simulink model "P2_SIL_Model_Diag"  (R2016a)
settings: Solver=ode2  StartTime=0.0  StopTime=Cycle_End  RelTol=1e-3
undefined symbols (not defined in the file): air, APP1_OOR, APP2_OOR, APP_Conversion_IN, APP_Mismatch, bms_inletair_temp, bms_maxchargecurrent, bms_maxdischargecurrent, BMS_Notfallkuehlung, BPP_Flt, cal, clt, ClutchEngag, CrankRequest, dcdc, eng, Engine, EngOverTemp, ENGTRQ_MSMCH_Degraded_CP, ENGTRQ_MSMCH_ErrCritical_CP, ENGTRQ_MSMCH_LimpHome_CP, EngTrqMismatch, env, ess, ESS, ESSOverTemp, fd, FFD, g, gb, Grade, IMG, KeyPos_Flt, KeyPosition, lib_APP_Conversion_IN, lib_ESS_plant_V1_2, lib_OBC_Manager, LossCAN, max_vehicle_rad_air_flow, MCUOverTemp, mot, MotDirMismatch, MotOverTemp, MotTrqMismatch, mph2kph, mph2ms, NeutralGear, obc, OBC_Manager, ParkGear, PRNDL_Flt, ReverseGear, RFD, rho, ShiftLeverPosition, sigbuilder_block, Speed, t_amb, time, tloop ... (+2)
libraries: simulink x104, EC2_libraries x12, Diagnostic x11, lib_CANerror_Detect x3, Utility x1
(part 6 of 11)

== system P2_SIL_Model_Diag/Controller/HSC/Camaro Fault Detection/Component Diagnostic/Driver Input Diagnostic ==
  note: Driver_CompStatus
      | 1 = Component Online
      | 0 = Component Offline
  note: APP1
      | APP2
      | BPP
      | Driver Component Status
      |
      | 1
      | 1
      | 1
      | 1
      |
      | 0
      | 1
      | 1
      | 1
      |
      | 1
      | 0
      | 1
      | 1
      |
      | 0
      | 0
      | 1
      | 0
      |
      | 1
      | 1
      | 0
      | 0
      |
      | 0
      | 0
      | 0
      | 0
  In1 : Inport
  Bus Creator : BusCreator  Inputs=1
  Bus Selector : BusSelector  OutputSignals=Driver_SigDiag.Drv_APP1_[%]_SigValid,Driver_SigDiag.Drv_APP2_[%]_SigValid,Driver_SigDiag.Drv_APP_Agree,Driver_SigDiag.Drv_BPP_[%]_SigValid,Driver_SigDiag.Drv_KeyPos_[0 3]_SigValid,Driver_SigDiag.Drv_PRNDL_SigValid
  Driver_Input_Diag : Stateflow chart  TreatAsAtomicUnit=on
  Logical Operator : Logic  Inputs=3  AllPortsSameDT=off  OutDataTypeStr=boolean
  Out1 : Outport
  wires:
  In1/1 -> Bus Selector/1
  Bus Selector/1 -> Logical Operator/1  "<Drv_APP1_[%]_SigValid>"
  Bus Selector/2 -> Logical Operator/2  "<Drv_APP2_[%]_SigValid>"
  Bus Selector/4 -> Driver_Input_Diag/2(Drv_BPP_SigValid)  "<Drv_BPP_[%]_SigValid>"
  Driver_Input_Diag/1(Driver_Input_Status) -> Bus Creator/1  "Driver_Input_Status"
  Logical Operator/1 -> Driver_Input_Diag/1(APP_Valid)  "APP_Valid"
  Bus Selector/3 -> Logical Operator/3  "<Drv_APP_Agree>"
  Bus Selector/5 -> Driver_Input_Diag/3(KeyPos)  "<Drv_KeyPos_[0 3]_SigValid>"
  Bus Creator/1 -> Out1/1
  Bus Selector/6 -> Driver_Input_Diag/4(PRNDL)  "<Drv_PRNDL_SigValid>"

== system P2_SIL_Model_Diag/Controller/HSC/Camaro Fault Detection/Component Diagnostic/ESS Component Diagnostic ==
  note: (Need modify)
  In1 : Inport
  BMS_CompDiag : Stateflow chart  Commented=on  TreatAsAtomicUnit=on
  BMS_CompDiag1 : Stateflow chart  TreatAsAtomicUnit=on
  Bus Creator : BusCreator  Inputs=1
  Bus Selector : BusSelector  OutputSignals=ESS_SigDiag.BMS_RollingAliveActive_SigValid,ESS_SigDiag.BMS_contactorsFailed_SigValid,ESS_SigDiag.BMS_essTemp_[degC]_SigValid,ESS_SigDiag.essTempRange[0_4],ESS_SigDiag.BMS_essSOC_0_1_SigValid,ESS_SigDiag.essTempRange[0_4],ESS_SigDiag.essCur_A_SigValid,ESS_SigDiag.BMSgdf_0_1,Driver_SigDiag.Drv_KeyPos_[0 3]_SigValid
  Compare To Zero : simulink/Logic and Bit Operations/Compare To Zero  relop===  OutDataTypeStr=boolean
  Data Type Conversion : DataTypeConversion
  HVessFltReset : Constant
  Logical Operator : Logic  Operator=OR  AllPortsSameDT=off  OutDataTypeStr=boolean
  Logical Operator1 : Logic  AllPortsSameDT=off  OutDataTypeStr=boolean
  Terminator : Terminator
  Terminator1 : Terminator
  Out1 : Outport
  wires:
  In1/1 -> Bus Selector/1
  Bus Selector/1 -> BMS_CompDiag1/1(BMS_RollingAliveActive_SigValid)  "<BMS_RollingAliveActive_SigValid>"
  Bus Selector/2 -> Logical Operator1/1, BMS_CompDiag1/2(BMS_contactorsFailed_SigValid)  "<BMS_contactorsFailed_SigValid>"
  Bus Creator/1 -> Out1/1
  BMS_CompDiag1/1(BMS_Status) -> Bus Creator/1  "BMS_Status"
  Bus Selector/4 -> Terminator/1  "<essTempRange[0_4]>"
  Bus Selector/3 -> Data Type Conversion/1  "<BMS_essTemp_[degC]_SigValid>"
  Data Type Conversion/1 -> BMS_CompDiag1/3(BMS_essTemp_SigValid)  "BMS_essTemp_SigValid"
  Bus Selector/5 -> BMS_CompDiag1/4(BMS_essSOC_0_1_SigValid)  "<BMS_essSOC_0_1_SigValid>"
  Bus Selector/6 -> Terminator1/1  "<essTempRange[0_4]>"
  Bus Selector/7 -> BMS_CompDiag1/5(essCur_A_SigValid)  "<essCur_A_SigValid>"
  Bus Selector/9 -> Compare To Zero/1  "<Drv_KeyPos_[0 3]_SigValid>"
  Compare To Zero/1 -> Logical Operator/1
  HVessFltReset/1 -> Logical Operator/2
  Logical Operator/1 -> BMS_CompDiag1/7(ClearFault)
  Bus Selector/8 -> Logical Operator1/2  "<BMSgdf_0_1>"
  Logical Operator1/1 -> BMS_CompDiag1/6(ess_GroundFault)

== system P2_SIL_Model_Diag/Controller/HSC/Camaro Fault Detection/Component Diagnostic/Engine Component Diagnostic ==
  note: Eng_Torq_MsmchLevel
      | 1:Normal torque
      | 2: Limit max power
      | 3: Deliver creep torque
      | 4: offline
  note: ENGTRQ_MSMCH_Degraded_CP (40Nm): ENGTRQ_Degraded fault code.
      | ENGTRQ_MSMCH_LimpHome_CP (70Nm): ENGTRQ_LimpHome
      | ENGTRQ_MSMCH_ErrCritical_CP (100Nm): ENGTRQ_ErrCritical
  note: Eng_tempRange
      | 1: normal
      | 2: high range
      | 3:above max
  note: add the temperature, mismatch torquesignal and have different status to the component
  note: 0: component needs to be offline
      | 1: component needs torque plant to deliver creep torque
      | 2: component needs torque plant to limit maximum torque delivery
      | 3: component needs torque plant to operate normally
  In1 : Inport
  Bus Creator : BusCreator  Inputs=1
  Bus Selector : BusSelector  OutputSignals=Engine_SigDiag.ECMRollingAliveActive,Engine_SigDiag.engTrqCmdRecvd_SigValid,Engine_SigDiag. ECMTrqCmd_Nm,Engine_SigDiag.EngActStdyStTorq_Nm,Engine_SigDiag.EngRunAtValid,Engine_SigDiag.Engine_Speed_rpm_SigValid,Engine_SigDiag.Eng_TempValid,Engine_SigDiag.Eng_TempRange[123],Driver_SigDiag.Drv_KeyPos_[0 3]_SigValid
  Bus Selector1 : BusSelector  OutputSignals=Eng_Torque_Mismch_Critical
  Compare To Zero : simulink/Logic and Bit Operations/Compare To Zero  relop===  OutDataTypeStr=boolean
  ECM_CompDiag : Stateflow chart  TreatAsAtomicUnit=on
  Eng_FltReset : Constant
  Eng_Torq_MsmchLevel : Stateflow chart  Commented=on  TreatAsAtomicUnit=on
  Logical Operator : Logic  Operator=OR  AllPortsSameDT=off  OutDataTypeStr=boolean
  Override  engTrqCmd : Subsystem
  Terminator1 : Terminator
  TorqMismatch Detection : Subsystem
  Out1 : Outport
  Out2 : Outport  Port=2
  wires:
  In1/1 -> Bus Selector/1
  Bus Selector/1 -> ECM_CompDiag/1(ECM_RollingAliveActive)  "<ECMRollingAliveActive>"
  Bus Selector/2 -> Override  engTrqCmd/1(In1)  "<engTrqCmdRecvd_SigValid>"
  Bus Selector/6 -> ECM_CompDiag/4(Engine_Speed_rpm_SigValid)  "<Engine_Speed_rpm_SigValid>"
  ECM_CompDiag/1(ECM_Status) -> Bus Creator/1  "ECM_Status"
  Compare To Zero/1 -> Logical Operator/1
  Eng_FltReset/1 -> Logical Operator/2
  Logical Operator/1 -> ECM_CompDiag/6(ClearFault)
  Bus Selector/9 -> Compare To Zero/1  "<Drv_KeyPos_[0 3]_SigValid>"
  Bus Selector/7 -> Terminator1/1  "<Eng_TempValid>"
  Bus Selector/8 -> ECM_CompDiag/5(Eng_TempRange_123)  "<Eng_TempRange[123]>"
  Bus Selector/3 -> TorqMismatch Detection/1(In1)  "< ECMTrqCmd_Nm>"
  Bus Selector/4 -> TorqMismatch Detection/2(In2)  "<EngActStdyStTorq_Nm>"
  Bus Selector/5 -> TorqMismatch Detection/3(In3)  "<EngRunAtValid>"
  Bus Creator/1 -> Out1/1
  TorqMismatch Detection/1(Eng_Torque_Mismch) -> Out2/1, Bus Selector1/1  "EngTrqMismchType"
  Bus Selector1/1 -> ECM_CompDiag/3(Eng_Torq_Msmch)  "<Eng_Torque_Mismch_Critical>"
  Override  engTrqCmd/1(Out1) -> ECM_CompDiag/2(engTrqCmdRecvd_SigValid)

== system P2_SIL_Model_Diag/Controller/HSC/Camaro Fault Detection/Component Diagnostic/Motor Component Diagnostic ==
  note: 0: component needs to be offline
      | 1: component needs torque plant to deliver creep torque
      | 2: component needs torque plant to limit maximum torque delivery
      | 3: component needs torque plant to operate normally
  In1 : Inport
  Bus Creator : BusCreator  Inputs=1
  Bus Selector : BusSelector  OutputSignals=Motor_SigDiag.MCURollingAliveActive,Motor_SigDiag.MCUTemp_degC_SigValid,Motor_SigDiag.MotorTemp_degC_SigValid,Motor_SigDiag.Motor_TrqCmd_Nm_SigValid,Motor_SigDiag.Torq_Feedback_Nm_SigValid,Motor_SigDiag.MCUTrqCmd_Nm,Motor_SigDiag.Torq_Feedback_Nm,Motor_SigDiag.Motor_Speed_rpm_SigValid,Motor_SigDiag.MCUTempRange[0_4],Motor_SigDiag.MotorTempRange[0_4],Motor_SigDiag.Direction_Command_SigValid,Motor_SigDiag.Direction_feedback_SigValid,Motor_SigDiag.Inverter_enable_state_SigValid,Motor_SigDiag.Direction_Command_0_1,Motor_SigDiag.Direction_feedback_0_1,Motor_SigDiag.Inverter_enable_state_0_1,Motor_SigDiag.DC_Bus_Voltage_SigValid,Motor_SigDiag.DC_Bus_Voltage_V,ESS_SigDiag. hvBattVolt_V
  Bus Selector1 : BusSelector  OutputSignals=MCU_Torque_Mismch_Critical
  MCU_CompDiag : Stateflow chart  TreatAsAtomicUnit=on
  MCU_ESS_Voltage_Mismatch : Subsystem
  Motor_Direction_Mismatch : Subsystem
  Override  fault : Subsystem  AncestorBlock=Diagnostic/Camaro Diagnostic/Input Conversions/DriverInput_Conversions/Override APP (%)
  Override  fault1 : Subsystem  AncestorBlock=Diagnostic/Camaro Diagnostic/Input Conversions/DriverInput_Conversions/Override APP (%)
  Terminator1 : Terminator
  Torque_Mismatch : Subsystem
  Out1 : Outport
  Out2 : Outport  Port=2
  wires:
  In1/1 -> Bus Selector/1
  MCU_CompDiag/1(MCU_Status) -> Bus Creator/1  "MCU_Status"
  Bus Selector/1 -> MCU_CompDiag/1(MCU_RollingAliveActive)  "<MCURollingAliveActive>"
  Bus Selector/2 -> MCU_CompDiag/2(MCUTemp_degC_SigValid)  "<MCUTemp_degC_SigValid>"
  Bus Selector/3 -> MCU_CompDiag/3(MotorTemp_degC_SigValid)  "<MotorTemp_degC_SigValid>"
  Bus Selector/4 -> MCU_CompDiag/4(Motor_TrqCmd_Nm_SigValid)  "<Motor_TrqCmd_Nm_SigValid>"
  Bus Selector/8 -> MCU_CompDiag/7(Motor_Speed_rpm_SigValid)  "<Motor_Speed_rpm_SigValid>"
  Bus Selector/9 -> MCU_CompDiag/8(MCUTempRange)  "<MCUTempRange[0_4]>"
  Bus Creator/1 -> Out1/1
  Bus Selector/13 -> Terminator1/1  "<Inverter_enable_state_SigValid>"
  Bus Selector/6 -> Torque_Mismatch/1(MCU_torq_command)  "<MCUTrqCmd_Nm>"
  Bus Selector/7 -> Torque_Mismatch/2(Torq_feedback)  "<Torq_Feedback_Nm>"
  Bus Selector/14 -> Motor_Direction_Mismatch/1(Direction_Command)  "<Direction_Command_0_1>"
  Bus Selector/15 -> Motor_Direction_Mismatch/2(Direction_Feedback)  "<Direction_feedback_0_1>"
  Bus Selector/16 -> Motor_Direction_Mismatch/3(Inverter_enable_state)  "<Inverter_enable_state_0_1>"
  Bus Selector/11 -> MCU_CompDiag/10(Dir_Command_SigValid)  "<Direction_Command_SigValid>"
  Bus Selector/12 -> MCU_CompDiag/11(Dir_feedback_SigValid)  "<Direction_feedback_SigValid>"
  Bus Selector/5 -> MCU_CompDiag/5(Torq_Feedback_SigValid)  "<Torq_Feedback_Nm_SigValid>"
  Bus Selector/17 -> MCU_CompDiag/13(dc_bus_voltage_SigValid)  "<DC_Bus_Voltage_SigValid>"
  Bus Selector/18 -> MCU_ESS_Voltage_Mismatch/1(MCU_Voltage)  "<DC_Bus_Voltage_V>"
  Bus Selector/19 -> MCU_ESS_Voltage_Mismatch/2(ESS_Voltage)  "< hvBattVolt_V>"
  MCU_ESS_Voltage_Mismatch/1(MCU_ESS_Voltage_Mismch) -> Override  fault/1(In1)
  Motor_Direction_Mismatch/1(Direction_Mismch) -> Override  fault1/1(In1)
  Torque_Mismatch/1(MCU_Torque_Mismch) -> Out2/1, Bus Selector1/1  "MCU_Torque_Mismch"
  Bus Selector1/1 -> MCU_CompDiag/6(MCU_torq_mismch)  "<MCU_Torque_Mismch_Critical>"
  Override  fault/1(Out1) -> MCU_CompDiag/14(Voltage_Mismch)
  Override  fault1/1(Out1) -> MCU_CompDiag/12(Dir_Mismch)
  Bus Selector/10 -> MCU_CompDiag/9(MotTempRange)  "<MotorTempRange[0_4]>"

== system P2_SIL_Model_Diag/Controller/HSC/Camaro Fault Detection/Component Diagnostic/Override Clutch Status ==
  note: This subsystem is used to override the model value of a signal to a constant value
  note: Override Switch Subsystem
  In1 : Inport
  Multiport Switch : MultiPortSwitch  DataPortOrder=Zero-based contiguous  Inputs=2  zeroidx=on
  Override Value : Constant  OutDataTypeStr=double
  Signal Override Switch 0 = Use Model 1 = Use Constant : Constant  Value=0
  Out1 : Outport
  wires:
  Signal Override Switch 0 = Use Model 1 = Use Constant/1 -> Multiport Switch/1
  In1/1 -> Multiport Switch/2
  Multiport Switch/1 -> Out1/1
  Override Value/1 -> Multiport Switch/3

== system P2_SIL_Model_Diag/Controller/HSC/Camaro Fault Detection/Component Diagnostic/Override Driver Status ==
  note: This subsystem is used to override the model value of a signal to a constant value
  note: Override Switch Subsystem
  In1 : Inport
  Multiport Switch : MultiPortSwitch  DataPortOrder=Zero-based contiguous  Inputs=2  zeroidx=on
  Override Value : Constant  Value=0  OutDataTypeStr=double
  Signal Override Switch 0 = Use Model 1 = Use Constant : Constant  Value=0
  Out1 : Outport
  wires:
  Signal Override Switch 0 = Use Model 1 = Use Constant/1 -> Multiport Switch/1
  In1/1 -> Multiport Switch/2
  Multiport Switch/1 -> Out1/1
  Override Value/1 -> Multiport Switch/3

== system P2_SIL_Model_Diag/Controller/HSC/Camaro Fault Detection/Component Diagnostic/Override ESS Status ==
  note: This subsystem is used to override the model value of a signal to a constant value
  note: Override Switch Subsystem
  In1 : Inport
  Multiport Switch : MultiPortSwitch  DataPortOrder=Zero-based contiguous  Inputs=2  zeroidx=on
  Override Value : Constant  Value=2  OutDataTypeStr=double
  Signal Override Switch 0 = Use Model 1 = Use Constant : Constant
  Out1 : Outport
  wires:
  Signal Override Switch 0 = Use Model 1 = Use Constant/1 -> Multiport Switch/1
  In1/1 -> Multiport Switch/2
  Multiport Switch/1 -> Out1/1
  Override Value/1 -> Multiport Switch/3

== system P2_SIL_Model_Diag/Controller/HSC/Camaro Fault Detection/Component Diagnostic/Override Engine Status ==
  note: This subsystem is used to override the model value of a signal to a constant value
  note: Override Switch Subsystem
  In1 : Inport
  Multiport Switch : MultiPortSwitch  DataPortOrder=Zero-based contiguous  Inputs=2  zeroidx=on
  Override Value : Constant  Value=2  OutDataTypeStr=double
  Signal Override Switch 0 = Use Model 1 = Use Constant : Constant
  Out1 : Outport
  wires:
  Signal Override Switch 0 = Use Model 1 = Use Constant/1 -> Multiport Switch/1
  In1/1 -> Multiport Switch/2
  Multiport Switch/1 -> Out1/1
  Override Value/1 -> Multiport Switch/3

== system P2_SIL_Model_Diag/Controller/HSC/Camaro Fault Detection/Component Diagnostic/Override MCU Status ==
  note: This subsystem is used to override the model value of a signal to a constant value
  note: Override Switch Subsystem
  In1 : Inport
  Multiport Switch : MultiPortSwitch  DataPortOrder=Zero-based contiguous  Inputs=2  zeroidx=on
  Override Value : Constant  Value=2  OutDataTypeStr=double
  Signal Override Switch 0 = Use Model 1 = Use Constant : Constant  Value=0
  Out1 : Outport
  wires:
  Signal Override Switch 0 = Use Model 1 = Use Constant/1 -> Multiport Switch/1
  In1/1 -> Multiport Switch/2
  Multiport Switch/1 -> Out1/1
  Override Value/1 -> Multiport Switch/3

== system P2_SIL_Model_Diag/Controller/HSC/Camaro Fault Detection/Component Diagnostic/Override TCM Status ==
  note: This subsystem is used to override the model value of a signal to a constant value
  note: Override Switch Subsystem
  In1 : Inport
  Multiport Switch : MultiPortSwitch  DataPortOrder=Zero-based contiguous  Inputs=2  zeroidx=on
  Override Value : Constant  Value=2  OutDataTypeStr=double
  Signal Override Switch 0 = Use Model 1 = Use Constant : Constant  Value=0
  Out1 : Outport
  wires:
  Signal Override Switch 0 = Use Model 1 = Use Constant/1 -> Multiport Switch/1
  In1/1 -> Multiport Switch/2
  Multiport Switch/1 -> Out1/1
  Override Value/1 -> Multiport Switch/3

== system P2_SIL_Model_Diag/Controller/HSC/Camaro Fault Detection/Component Diagnostic/Transmission Component Diagnostic ==
  In1 : Inport
  Bus Creator : BusCreator  Inputs=1
  Bus Selector : BusSelector  OutputSignals=Transmission_SigDiag.TCMRollingAliveActive_SigValid,Transmission_SigDiag.LvrPosTrnsShft_SigValid,Transmission_SigDiag.TransEstGear_SigValid,Transmission_SigDiag.LockupCmd_SigValid
  TCM_CompDia : Stateflow chart  TreatAsAtomicUnit=on
  Out1 : Outport
  wires:
  In1/1 -> Bus Selector/1
  Bus Creator/1 -> Out1/1  "TCM_Status"
  Bus Selector/1 -> TCM_CompDia/1(TCMRollingAliveActive_SigValid)  "<TCMRollingAliveActive_SigValid>"
  Bus Selector/2 -> TCM_CompDia/2(LvrPosTrnsShft_SigValid)  "<LvrPosTrnsShft_SigValid>"
  Bus Selector/3 -> TCM_CompDia/3(TransEstGear_SigValid)  "<TransEstGear_SigValid>"
  Bus Selector/4 -> TCM_CompDia/4(LockupCmd_SigValid)  "<LockupCmd_SigValid>"
  TCM_CompDia/1(TCM_Status) -> Bus Creator/1  "TCM_Status"

== system P2_SIL_Model_Diag/Controller/HSC/Camaro Fault Detection/Input Conversions/BMS_Conversions ==
  note: BMS: Conversions and Override Switches
      | (Battery Management System)
  In1 : Inport
  BMS_rollingAliveCnt : Subsystem  Commented=on
  Bus Creator : BusCreator  Inputs=9
  Bus Selector : BusSelector  OutputSignals=from_CAN.fromHV_CAN.from_BMSHybrid.RollingAliveCnt,from_CAN.fromHV_CAN.from_BMSHybrid.BMS_HYB_02.MO_BMS_Sollmodus,from_CAN.fromHV_CAN.from_BMSHybrid.BMS_HYB_02.BMS_IstModus,from_CAN.fromHV_CAN.from_BMSHybrid.BMS_HYB_02.BMS_IstStrom,from_CAN.fromHV_CAN.from_BMSHybrid.BMS_SOC,from_CAN.fromHV_CAN.from_BMSHybrid.BMS_HYB_02.BMS_IstSpannung,from_CAN.fromHV_CAN.from_BMSHybrid.BMS_Spannung_ZwKr,from_CAN.fromHV_CAN.from_BMSHybrid.BMS_HYB_06.BMS_Temperatur,from_CAN.fromHV_CAN.from_BMSHybrid.BMS_HYB_02.BMS_Fehler_Isolation
  Conversion  BMS_gdf : DataTypeConversion  OutDataTypeStr=boolean
  Conversion  closeContactorsCmd : DataTypeConversion  OutDataTypeStr=boolean
  Conversion  contactorsClsd : DataTypeConversion  OutDataTypeStr=boolean
  Conversion  essTemp_K : DataTypeConversion  OutDataTypeStr=double
  Conversion  hvBattVolt_V : DataTypeConversion  OutDataTypeStr=double
  Conversion  hvBusVolt_V : DataTypeConversion  OutDataTypeStr=double
  Conversion  rollingAliveCnt : DataTypeConversion  OutDataTypeStr=int8
  Conversion essCur_A : DataTypeConversion  OutDataTypeStr=double
  Conversion essSOC_0_1 : DataTypeConversion  OutDataTypeStr=double
  K to C : Bias  Bias=-273.15
  Override  BMS_gdf 0_1 : Subsystem
  Override  closeContactorsCmd : Subsystem
  Override  contactorsClsd : Subsystem
  Override  essCur_A : Subsystem
  Override  essSOC_0_1 : Subsystem
  Override  essTemp_C : Subsystem
  Override  hvBattVolt_V : Subsystem
  Override  hvBusVolt_V : Subsystem
  Override  rollingAliveCnt [1_3] : Subsystem
  Out1 : Outport
  wires:
  In1/1 -> Bus Selector/1
  Conversion  rollingAliveCnt/1 -> Override  rollingAliveCnt [1_3]/1(In1)
  Override  rollingAliveCnt [1_3]/1(Out1) -> Bus Creator/1  "BMSrollingAliveCnt [123]"
  Bus Creator/1 -> Out1/1  "BMS_Conv"
  Conversion  closeContactorsCmd/1 -> Override  closeContactorsCmd/1(In1)
  Override  closeContactorsCmd/1(Out1) -> Bus Creator/2  "closeContactorsCmd [01]"
  Conversion  contactorsClsd/1 -> Override  contactorsClsd/1(In1)
  Conversion essCur_A/1 -> Override  essCur_A/1(In1)
  Conversion essSOC_0_1/1 -> Override  essSOC_0_1/1(In1)
  Conversion  hvBattVolt_V/1 -> Override  hvBattVolt_V/1(In1)
  Conversion  hvBusVolt_V/1 -> Override  hvBusVolt_V/1(In1)
  Override  contactorsClsd/1(Out1) -> Bus Creator/3  "contactorsClsd"
  Override  essSOC_0_1/1(Out1) -> Bus Creator/5  "essSOC_0_1"
  Override  hvBattVolt_V/1(Out1) -> Bus Creator/6  "hvBattVolt_V"
  Override  essCur_A/1(Out1) -> Bus Creator/4  "essCur_A"
  Override  hvBusVolt_V/1(Out1) -> Bus Creator/7  "hvBusVolt_V"
  Conversion  essTemp_K/1 -> K to C/1
  Override  essTemp_C/1(Out1) -> Bus Creator/8  "essTemp_C"
  K to C/1 -> Override  essTemp_C/1(In1)
  Conversion  BMS_gdf/1 -> Override  BMS_gdf 0_1/1(In1)
  Override  BMS_gdf 0_1/1(Out1) -> Bus Creator/9  "BMS_gdf"
  Bus Selector/3 -> Conversion  contactorsClsd/1  "<BMS_IstModus>"
  Bus Selector/8 -> Conversion  essTemp_K/1  "<BMS_Temperatur>"
  Bus Selector/9 -> Conversion  BMS_gdf/1  "<BMS_Fehler_Isolation>"
  Bus Selector/6 -> Conversion  hvBattVolt_V/1  "<BMS_IstSpannung>"
  Bus Selector/5 -> Conversion essSOC_0_1/1  "<BMS_SOC>"
  Bus Selector/4 -> Conversion essCur_A/1  "<BMS_IstStrom>"
  Bus Selector/1 -> Conversion  rollingAliveCnt/1  "<RollingAliveCnt>"
  Bus Selector/7 -> Conversion  hvBusVolt_V/1  "<BMS_Spannung_ZwKr>"
  Bus Selector/2 -> Conversion  closeContactorsCmd/1  "<MO_BMS_Sollmodus>"

== system P2_SIL_Model_Diag/Controller/HSC/Camaro Fault Detection/Input Conversions/Clutch_Conversions ==
  note: Clutch: Input Conversions and Override Switches
  In1 : Inport
  Bus Creator : BusCreator  Inputs=3
  Bus Selector : BusSelector  OutputSignals=from_CAN.fromHV_CAN.from_MCU.EngageClutch,from_CAN.fromHV_CAN.from_MCU.clt_plant_spd_in
  Clutch_Rolling : Subsystem
  Conversion  Engage_Clutch : DataTypeConversion  OutDataTypeStr=boolean
  Conversion  clt_plant_spd_out : DataTypeConversion  OutDataTypeStr=double
  Conversion  rollingAliveCnt : DataTypeConversion  OutDataTypeStr=int8
  "Override  Engage_Clutch " : Subsystem  AncestorBlock="Diagnostic/Camaro Diagnostic/Input Conversions/MCU_Conversions/Override  rollingAliveCnt [123]"
  Override  clt_plant_spd_out : Diagnostic/Camaro Diagnostic/Input Conversions/MCU_Conversions/Override  rollingAliveCnt [123]
  Override  rollingAliveCnt [123] : Subsystem
  Out1 : Outport
  wires:
  In1/1 -> Bus Selector/1
  Conversion  rollingAliveCnt/1 -> Override  rollingAliveCnt [123]/1(In1)
  Override  rollingAliveCnt [123]/1(Out1) -> Bus Creator/1  "ClutchrollingAliveCnt [123]"
  Bus Creator/1 -> Out1/1  "Clutch_Conv"
  Bus Selector/1 -> Conversion  Engage_Clutch/1  "<EngageClutch>"
  "Override  Engage_Clutch "/1(Out1) -> Bus Creator/2  "Engage_Clutch"
  Conversion  Engage_Clutch/1 -> "Override  Engage_Clutch "/1(In1)
  Conversion  clt_plant_spd_out/1 -> Override  clt_plant_spd_out/1
  Override  clt_plant_spd_out/1 -> Bus Creator/3  "clt_plant_spd_out"
  Clutch_Rolling/1(Out1) -> Conversion  rollingAliveCnt/1
  Bus Selector/2 -> Conversion  clt_plant_spd_out/1  "<clt_plant_spd_in>"

== system P2_SIL_Model_Diag/Controller/HSC/Camaro Fault Detection/Input Conversions/DriverInput_Conversions ==
  note: SysPwrMd (EC3)
      | 0 - Off
      | 1 -  Accessory
      | 2 - Run
      | 3 - Crank Request
  note: Driver Controls: Conversions and Override Switches
  In1 : Inport
  Bus Creator : BusCreator  Inputs=6
  Bus Selector : BusSelector  OutputSignals=from_Analog.Com_APP.APP_Norm_Pos1,from_Analog.Com_APP.APP_Norm_Pos2,from_Analog.drv_BPP_req_[%],from_Analog.KeyPos,from_Analog.ShiftLvrPos,from_CAN.fromEBCAN.from_ECM.VehSpdAvgDrvn
  Conversion  APP1 (%) : DataTypeConversion  OutDataTypeStr=double
  Conversion  APP2 (%) : DataTypeConversion  OutDataTypeStr=double
  Conversion  BPP (%) : DataTypeConversion  OutDataTypeStr=double
  Conversion  KeyPos [0_3] : DataTypeConversion  OutDataTypeStr=int8
  Conversion  V [mph] : DataTypeConversion  OutDataTypeStr=double
  Conversion PRNDL : DataTypeConversion  OutDataTypeStr=uint8
  Gain : Gain  Gain=-1
  Override  KeyPos [0_3] : Subsystem
  Override APP (%) : Subsystem
  Override APP (%)1 : Diagnostic/Camaro Diagnostic/Input Conversions/DriverInput_Conversions/Override APP (%)
  Override BPP (%) : Subsystem
  Override PRNDL : Subsystem
  Override V [mph] : Subsystem
  Out1 : Outport
  wires:
  In1/1 -> Bus Selector/1
  Conversion  APP1 (%)/1 -> Override APP (%)/1(In1)
  Override APP (%)/1(Out1) -> Bus Creator/1  "APP1 [%]"
  Bus Selector/1 -> Conversion  APP1 (%)/1  "<APP_Norm_Pos1>"
  Bus Selector/3 -> Conversion  BPP (%)/1  "<drv_BPP_req_[%]>"
  Bus Selector/4 -> Conversion  KeyPos [0_3]/1  "<KeyPos>"
  Conversion  KeyPos [0_3]/1 -> Override  KeyPos [0_3]/1(In1)
  Override BPP (%)/1(Out1) -> Bus Creator/3  "BPP [%]"
  Override  KeyPos [0_3]/1(Out1) -> Bus Creator/4  "keyPos [0_3]"
  Bus Creator/1 -> Out1/1  "DriverControls_Conv"
  Conversion  BPP (%)/1 -> Gain/1
  Gain/1 -> Override BPP (%)/1(In1)
  Conversion PRNDL/1 -> Override PRNDL/1(In1)
  Override PRNDL/1(Out1) -> Bus Creator/5  "PRNDL"
  Bus Selector/2 -> Conversion  APP2 (%)/1  "<APP_Norm_Pos2>"
  Bus Selector/5 -> Conversion PRNDL/1  "<ShiftLvrPos>"
  Override APP (%)1/1 -> Bus Creator/2  "APP2[%]"
  Conversion  APP2 (%)/1 -> Override APP (%)1/1
  Bus Selector/6 -> Conversion  V [mph]/1  "<VehSpdAvgDrvn>"
  Conversion  V [mph]/1 -> Override V [mph]/1(In1)
  Override V [mph]/1(Out1) -> Bus Creator/6  "V [mph]"

== system P2_SIL_Model_Diag/Controller/HSC/Camaro Fault Detection/Input Conversions/ECM_Conversions ==
  note: ECM: Input Conversions and Override Switches
      | (Engine and ECM)
  In1 : Inport
  Bus Creator : BusCreator  Inputs=6
  Bus Selector : BusSelector  OutputSignals=from_CAN.fromEBCAN.from_ECM.ECM_RollingAliveCnt,from_CAN.fromEBCAN.from_ECM.EngTrqCmd,from_CAN.fromEBCAN.from_ECM.EngSpd_RPM,from_CAN.fromEBCAN.from_ECM.Eng_Temp,from_CAN.fromEBCAN.from_ECM.EngRunAtv,from_CAN.fromEBCAN.from_ECM.EngActStdyStTorq
  Conversion  ECMTrqCmd_Nm : DataTypeConversion  OutDataTypeStr=double
  Conversion  EngActStdyStTorq_Nm : DataTypeConversion  OutDataTypeStr=double
  Conversion  EngRunAtv : DataTypeConversion  OutDataTypeStr=boolean
  Conversion  Engine_Speed_rpm : DataTypeConversion  OutDataTypeStr=double
  Conversion  Engine_Temp[DegC] : DataTypeConversion  OutDataTypeStr=double
  Conversion  rollingAliveCnt : DataTypeConversion  OutDataTypeStr=int8
  Override  ECMTrqCmd_Nm : Diagnostic/Camaro Diagnostic/Input Conversions/MCU_Conversions/Override  rollingAliveCnt [123]
  Override  ECMrollingAliveCnt : Subsystem
  Override  EngActStdyStTorq_Nm : Subsystem
  Override  EngRunAtv : Subsystem
  Override  EngineSpeed_rpm : Diagnostic/Camaro Diagnostic/Input Conversions/MCU_Conversions/Override  rollingAliveCnt [123]
  Override  Engine_Temp[DegC] : Subsystem
  Out1 : Outport
  wires:
  In1/1 -> Bus Selector/1
  Conversion  rollingAliveCnt/1 -> Override  ECMrollingAliveCnt/1(In1)
  Override  ECMrollingAliveCnt/1(Out1) -> Bus Creator/1  "ECMrollingAliveCnt [123]"
  Bus Creator/1 -> Out1/1  "ECM_Conv"
  Bus Selector/2 -> Conversion  ECMTrqCmd_Nm/1  "<EngTrqCmd>"
  Override  ECMTrqCmd_Nm/1 -> Bus Creator/2  "ECMTrqCmd_Nm"
  Conversion  ECMTrqCmd_Nm/1 -> Override  ECMTrqCmd_Nm/1
  Bus Selector/3 -> Conversion  Engine_Speed_rpm/1  "<EngSpd_RPM>"
  Conversion  Engine_Speed_rpm/1 -> Override  EngineSpeed_rpm/1
  Override  EngineSpeed_rpm/1 -> Bus Creator/3  "EngineSpeed_rpm"
  Bus Selector/4 -> Conversion  Engine_Temp[DegC]/1  "<Eng_Temp>"
  Bus Selector/5 -> Conversion  EngRunAtv/1  "<EngRunAtv>"
  Bus Selector/6 -> Conversion  EngActStdyStTorq_Nm/1  "<EngActStdyStTorq>"
  Conversion  Engine_Temp[DegC]/1 -> Override  Engine_Temp[DegC]/1(In1)
  Conversion  EngRunAtv/1 -> Override  EngRunAtv/1(In1)
  Conversion  EngActStdyStTorq_Nm/1 -> Override  EngActStdyStTorq_Nm/1(In1)
  Override  Engine_Temp[DegC]/1(Out1) -> Bus Creator/4  "Engine_Temp[DegC]"
  Override  EngRunAtv/1(Out1) -> Bus Creator/5  "EngRunAtv"
  Override  EngActStdyStTorq_Nm/1(Out1) -> Bus Creator/6  "EngActStdyStTorq_Nm"
  Bus Selector/1 -> Conversion  rollingAliveCnt/1  "<ECM_RollingAliveCnt>"

== system P2_SIL_Model_Diag/Controller/HSC/Camaro Fault Detection/Input Conversions/MCU_Conversions ==
  note: MCU: Input Conversions and Override Switches
      | (Motor Control Unit)
  In1 : Inport
  Bus Creator : BusCreator  Inputs=10
  Bus Selector : BusSelector  OutputSignals=from_CAN.fromHV_CAN.from_MCU.RollingAliveCnt,from_CAN.fromHV_CAN.from_MCU.mcu_temp,from_CAN.fromHV_CAN.from_MCU.mot_temp,from_CAN.fromHV_CAN.from_MCU.Torque_Command,from_CAN.fromHV_CAN.from_MCU.D2_Torque_Feedback,from_CAN.fromHV_CAN.from_MCU.D2_Motor_Speed,from_CAN.fromHV_CAN.from_MCU.D2_Torque_Feedback,from_CAN.fromHV_CAN.from_MCU.D6_Inverter_Enable_State,from_CAN.fromHV_CAN.from_MCU.D1_DC_Bus_Voltage
  Constant : Constant
  Constant1 : Constant
  Conversion  DC_Bus_Voltage : DataTypeConversion  OutDataTypeStr=double
  Conversion  Direction_feedback : DataTypeConversion  OutDataTypeStr=boolean
  Conversion  Inverter_enable_state : DataTypeConversion  OutDataTypeStr=boolean
  Conversion  MCUTemp_C : DataTypeConversion  OutDataTypeStr=double
  Conversion  MCUTrqCmd_Nm : DataTypeConversion  OutDataTypeStr=double
  Conversion  MotorSpeed_rpm : DataTypeConversion  OutDataTypeStr=double
  Conversion  MotorTemp_C : DataTypeConversion  OutDataTypeStr=double
  Conversion  Motor_Direction : DataTypeConversion  OutDataTypeStr=boolean
  Conversion  Torq_Feedback : DataTypeConversion  OutDataTypeStr=double
  Conversion  rollingAliveCnt : DataTypeConversion  OutDataTypeStr=int8
  Override  DC_Bus_Voltage : Subsystem
  Override  Direction_feedback : Subsystem
  Override  Inverter_enable_state : Subsystem
  "Override  MCUTemp_C " : Diagnostic/Camaro Diagnostic/Input Conversions/MCU_Conversions/Override  rollingAliveCnt [123]
  Override  MCUTrqCmd_Nm : Diagnostic/Camaro Diagnostic/Input Conversions/MCU_Conversions/Override  rollingAliveCnt [123]
  Override  MotorSpeed_rpm : Diagnostic/Camaro Diagnostic/Input Conversions/MCU_Conversions/Override  rollingAliveCnt [123]
  Override  MotorTemp_C : Diagnostic/Camaro Diagnostic/Input Conversions/MCU_Conversions/Override  rollingAliveCnt [123]
  Override  Motor_Direction : Subsystem
  Override  Torq_Feedback : Subsystem
  Override  rollingAliveCnt [123] : Subsystem
  Terminator3 : Terminator
  Out1 : Outport
  wires:
  In1/1 -> Bus Selector/1
  Conversion  rollingAliveCnt/1 -> Override  rollingAliveCnt [123]/1(In1)
  Override  rollingAliveCnt [123]/1(Out1) -> Bus Creator/1  "MCUrollingAliveCnt [123]"
  Bus Creator/1 -> Out1/1  "MCU_Conv"
  "Override  MCUTemp_C "/1 -> Bus Creator/2  "MCUTemp_C"
  Conversion  MCUTemp_C/1 -> "Override  MCUTemp_C "/1
  Bus Selector/3 -> Conversion  MotorTemp_C/1  "<mot_temp>"
  Conversion  MotorTemp_C/1 -> Override  MotorTemp_C/1
  Override  MotorTemp_C/1 -> Bus Creator/3  "Motor_Temp_C"
  Bus Selector/4 -> Conversion  MCUTrqCmd_Nm/1  "<Torque_Command>"
  Conversion  MCUTrqCmd_Nm/1 -> Override  MCUTrqCmd_Nm/1
  Override  MCUTrqCmd_Nm/1 -> Bus Creator/4  "MCUTrqCmd_Nm"
  Bus Selector/6 -> Conversion  MotorSpeed_rpm/1  "<D2_Motor_Speed>"
  Conversion  MotorSpeed_rpm/1 -> Override  MotorSpeed_rpm/1
  Override  MotorSpeed_rpm/1 -> Bus Creator/6  "MotorSpeed_rpm"
  Bus Selector/5 -> Conversion  Torq_Feedback/1  "<D2_Torque_Feedback>"
  Conversion  Torq_Feedback/1 -> Override  Torq_Feedback/1(In1)
  Override  Torq_Feedback/1(Out1) -> Bus Creator/5  "Torq_Feedback_Nm"
  Conversion  Motor_Direction/1 -> Override  Motor_Direction/1(In1)
  Override  Motor_Direction/1(Out1) -> Bus Creator/7  "Direction_Command_0_1"
  Bus Selector/8 -> Conversion  Inverter_enable_state/1  "<D6_Inverter_Enable_State>"
  Conversion  Direction_feedback/1 -> Override  Direction_feedback/1(In1)
  Conversion  Inverter_enable_state/1 -> Override  Inverter_enable_state/1(In1)
  Override  Direction_feedback/1(Out1) -> Bus Creator/8  "Direction_feedback_0_1"
  Override  Inverter_enable_state/1(Out1) -> Bus Creator/9  "Inverter_enable_state_0_1"
  Bus Selector/9 -> Conversion  DC_Bus_Voltage/1  "<D1_DC_Bus_Voltage>"
  Conversion  DC_Bus_Voltage/1 -> Override  DC_Bus_Voltage/1(In1)
  Override  DC_Bus_Voltage/1(Out1) -> Bus Creator/10  "DC_Bus_Voltage_V"
  Constant/1 -> Conversion  Direction_feedback/1
  Constant1/1 -> Conversion  Motor_Direction/1
  Bus Selector/1 -> Conversion  rollingAliveCnt/1  "<RollingAliveCnt>"
  Bus Selector/2 -> Conversion  MCUTemp_C/1  "<mcu_temp>"
  Bus Selector/7 -> Terminator3/1  "<D2_Torque_Feedback>"

== system P2_SIL_Model_Diag/Controller/HSC/Camaro Fault Detection/Input Conversions/TCM_Conversions ==
  note: TCM: Input Conversions and Override Switches
      | (Transmission Control Module)
  In1 : Inport
  Bus Creator : BusCreator  Inputs=4
  Bus Selector : BusSelector  OutputSignals=from_CAN.fromVEH_CAN.from_TCM.TrnsShftLvrPos,from_CAN.fromVEH_CAN.from_TCM.TransEstGear,from_CAN.fromVEH_CAN.from_TCM.LockupCmd
  Conversion  LockupCmd : DataTypeConversion  OutDataTypeStr=boolean
  Conversion  LvrPosTrnsShft : DataTypeConversion  OutDataTypeStr=int8
  Conversion  TransEstGear : DataTypeConversion  OutDataTypeStr=int8
  Conversion  rollingAliveCnt : DataTypeConversion  OutDataTypeStr=int8
  Override  LockupCmd : Diagnostic/Camaro Diagnostic/Input Conversions/MCU_Conversions/Override  rollingAliveCnt [123]
  "Override  LvrPosTrnsShft " : Diagnostic/Camaro Diagnostic/Input Conversions/MCU_Conversions/Override  rollingAliveCnt [123]
  Override  TransEstGear : Diagnostic/Camaro Diagnostic/Input Conversions/MCU_Conversions/Override  rollingAliveCnt [123]
  Override  rollingAliveCnt [123] : Subsystem
  TCM_Rolling : Subsystem
  Out1 : Outport
  wires:
  Override  LockupCmd/1 -> Bus Creator/4  "LockupCmd_0_1"
  Conversion  LockupCmd/1 -> Override  LockupCmd/1
  Bus Selector/3 -> Conversion  LockupCmd/1  "<LockupCmd>"
  Override  TransEstGear/1 -> Bus Creator/3  "TransEstGear"
  Conversion  TransEstGear/1 -> Override  TransEstGear/1
  Bus Selector/2 -> Conversion  TransEstGear/1  "<TransEstGear>"
  Conversion  LvrPosTrnsShft/1 -> "Override  LvrPosTrnsShft "/1
  "Override  LvrPosTrnsShft "/1 -> Bus Creator/2  "LvrPosTrnsShft"
  Bus Selector/1 -> Conversion  LvrPosTrnsShft/1  "<TrnsShftLvrPos>"
  Bus Creator/1 -> Out1/1  "TCM_Conv"
  Override  rollingAliveCnt [123]/1(Out1) -> Bus Creator/1  "TCMrollingAliveCnt [123]"
  Conversion  rollingAliveCnt/1 -> Override  rollingAliveCnt [123]/1(In1)
  In1/1 -> Bus Selector/1
  TCM_Rolling/1(Out1) -> Conversion  rollingAliveCnt/1

== system P2_SIL_Model_Diag/Controller/HSC/Camaro Fault Detection/Signal Diagnostic/Clutch Signal Diagnostic ==
  note: 0: success
      | 1: Engage failed
  Sensors1 : Inport
  Bus Creator : BusCreator  Inputs=4
  Bus Selector : BusSelector  OutputSignals=Clutch_Conv.ClutchrollingAliveCnt [123],Clutch_Conv.Engage_Clutch,Clutch_Conv.clt_plant_spd_out
  Compare To Constant : simulink/Logic and Bit Operations/Compare To Constant  relop===  const=1  OutDataTypeStr=boolean
  Compare To Zero : simulink/Logic and Bit Operations/Compare To Zero  relop=>  OutDataTypeStr=boolean
  Interval Test : simulink/Logic and Bit Operations/Interval Test  IntervalClosedRight=on  uplimit=1  IntervalClosedLeft=on  lowlimit=0  OutDataTypeStr=boolean
  Interval Test2 : simulink/Logic and Bit Operations/Interval Test  IntervalClosedRight=on  uplimit=8000  IntervalClosedLeft=on  lowlimit=0  OutDataTypeStr=boolean
  Logical Operator : Logic  Operator=NXOR  IconShape=distinctive  AllPortsSameDT=off  OutDataTypeStr=boolean
  Logical Operator1 : Logic  Operator=NOT  AllPortsSameDT=off  OutDataTypeStr=boolean
  Override  Engage : Subsystem  AncestorBlock=Diagnostic/Camaro Diagnostic/Input Conversions/DriverInput_Conversions/Override APP (%)
  Rolling Alive Counter Detection : Subsystem  AncestorBlock=Diagnostic/Camaro Diagnostic/Signal Diagnostic/Motor Signal Diagnostic/Rolling Alive Counter Detection
  Out2 : Outport
  wires:
  Sensors1/1 -> Bus Selector/1
  Bus Selector/1 -> Rolling Alive Counter Detection/1(In1)  "<ClutchrollingAliveCnt [123]>"
  Bus Selector/2 -> Compare To Constant/1, Interval Test/1  "<Engage_Clutch>"
  Bus Selector/3 -> Interval Test2/1, Compare To Zero/1  "<clt_plant_spd_out>"
  Bus Creator/1 -> Out2/1
  Interval Test/1 -> Bus Creator/2  "Engage_Clutch_SigValid"
  Rolling Alive Counter Detection/1(Out1) -> Bus Creator/1  "ClutchRollingAliveActive"
  Interval Test2/1 -> Bus Creator/4  "clt_plant_spd_out_SigValid"
  Compare To Zero/1 -> Logical Operator/2
  Compare To Constant/1 -> Logical Operator/1
  Logical Operator/1 -> Logical Operator1/1
  Logical Operator1/1 -> Override  Engage/1(In1)  "Engage_Failed"
  Override  Engage/1(Out1) -> Bus Creator/3  "Engage_Failed"

== system P2_SIL_Model_Diag/Controller/HSC/Camaro Fault Detection/Signal Diagnostic/Driver Signal Diagnostic ==
  note: L: out of combination?
  note: PRNDL
  note: Driver Controls : Signal Diagnostic
  Sensors1 : Inport
  APP_Crosscheck : Subsystem
  AccPedalValidity : Stateflow chart  TreatAsAtomicUnit=on
  AccPedalValidity1 : Stateflow chart  TreatAsAtomicUnit=on
  Braking fail to decelerate : Subsystem
  Bus Creator : BusCreator  Inputs=7
  Bus Selector : BusSelector  OutputSignals=DriverControls_Conv.APP1 [%],DriverControls_Conv.APP2[%],DriverControls_Conv.BPP [%],DriverControls_Conv. keyPos [0_3],DriverControls_Conv.PRNDL
  Constant : Constant  Value=0
  Constant1 : Constant  Value=0
  Constant3 : Constant
  Conversion  APP1 (%) : DataTypeConversion  OutDataTypeStr=boolean
  Interval Test : simulink/Logic and Bit Operations/Interval Test  IntervalClosedRight=on  uplimit=0  IntervalClosedLeft=on  lowlimit=-100  OutDataTypeStr=boolean
  Interval Test1 : simulink/Logic and Bit Operations/Interval Test  IntervalClosedRight=on  uplimit=3  IntervalClosedLeft=on  lowlimit=0  OutDataTypeStr=boolean
  Interval Test2 : simulink/Logic and Bit Operations/Interval Test  IntervalClosedRight=on  uplimit=4  IntervalClosedLeft=on  lowlimit=0  OutDataTypeStr=boolean
  Latch : Subsystem
  Driver_SigDiag : Outport
  wires:
  Sensors1/1 -> Bus Selector/1
  Bus Selector/1 -> APP_Crosscheck/1(In1), AccPedalValidity/2(signalValue)  "<APP1 [%]>"
  Bus Selector/2 -> APP_Crosscheck/2(In2), AccPedalValidity1/2(signalValue)  "<APP2[%]>"
  Constant/1 -> AccPedalValidity/1(clearFaults)
  Constant1/1 -> AccPedalValidity1/1(clearFaults)
  Bus Selector/3 -> Braking fail to decelerate/1(In1), Braking fail to decelerate/2(In2), Interval Test/1  "<BPP [%]>"
  Bus Selector/4 -> Interval Test1/1  "< keyPos [0_3]>"
  AccPedalValidity/1(signalValid) -> Bus Creator/1  "Drv_APP1_[%]_SigValid"
  Interval Test/1 -> Bus Creator/4  "Drv_BPP_[%]_SigValid"
  Interval Test1/1 -> Bus Creator/6  "Drv_KeyPos_[0 3]_SigValid"
  AccPedalValidity1/1(signalValid) -> Bus Creator/2  "Drv_APP2_[%]_SigValid"
  Bus Creator/1 -> Driver_SigDiag/1  "Driver_SignalDiag"
  Bus Selector/5 -> Interval Test2/1  "<PRNDL>"
  Interval Test2/1 -> Bus Creator/7  "Drv_PRNDL_SigValid"
  Constant3/1 -> Conversion  APP1 (%)/1
  Conversion  APP1 (%)/1 -> Latch/2(In2)
  APP_Crosscheck/1(Out1) -> Latch/1(In1)  "Drv_APP_Agree"
  Latch/1(Out1) -> Bus Creator/3  "Drv_APP_Agree"
  Braking fail to decelerate/1(Out1) -> Bus Creator/5  "Brake_Failed"

== system P2_SIL_Model_Diag/Controller/HSC/Camaro Fault Detection/Signal Diagnostic/ESS Signal Diagnostic ==
  note: //add SOC and current checks//
  note: Temperature Range check :
      | 0 = below normal operation (<-28)
      | 1 = low range (<0 - >-28)
      | 2 = normal range (0 -30 C)
      | 3= high range (>30)
      | 4= above max value allowed (>55)
  note: SOC Range check definition :
      | 0 = below normal operation (<0.15)
      | 1 = low range ([0.15 0.30])
      | 2 = normal range (0.3)
      | 3= SOC high/full (>0.95)
  note: 1) Rolling alive detection : is the component on and transmitting?
      | 2) Probably move the voltage check to component diagnostic (no signal from Bosch to check the contactors status)
      | 3) Is  the T signal within an acceptable range?
  note: BMS : Signal Diagnostic
  Sensors1 : Inport
  " " : simulink/Logic and Bit Operations/Compare To Constant  relop=>  const=0.5  OutDataTypeStr=boolean
  Abs : Abs
  Bus Creator : BusCreator  Inputs=9
  Bus Selector : BusSelector  OutputSignals=BMS_Conv. BMSrollingAliveCnt [123],BMS_Conv. hvBattVolt_V,BMS_Conv.hvBusVolt_V,BMS_Conv.essTemp_C,BMS_Conv.essSOC_0_1,BMS_Conv.essCur_A,BMS_Conv.BMS_gdf
  Constant : Constant
  Constant1 : Constant
  Interval Test : simulink/Logic and Bit Operations/Interval Test  IntervalClosedRight=on  uplimit=180  IntervalClosedLeft=on  lowlimit=-315  OutDataTypeStr=boolean
  Interval Test1 : simulink/Logic and Bit Operations/Interval Test  IntervalClosedRight=on  uplimit=1  IntervalClosedLeft=on  lowlimit=0  OutDataTypeStr=boolean
  Rolling Alive Counter Detection : Subsystem
  Sum : Sum  Inputs=+-
  essSOCValidity_Check : Subsystem
  essSOC_0_1Range : Stateflow chart  TreatAsAtomicUnit=on
  essTsignalRange : Stateflow chart  TreatAsAtomicUnit=on
  essTsignalValidity_Check : Subsystem
  ESS_SigDiag : Outport
  wires:
  Sensors1/1 -> Bus Selector/1
  Bus Selector/1 -> Rolling Alive Counter Detection/1(In1)  "< BMSrollingAliveCnt [123]>"
  Rolling Alive Counter Detection/1(Out1) -> Bus Creator/1  "BMS_RollingAliveActive_SigValid"
  Bus Selector/2 -> Bus Creator/3, Sum/1  "< hvBattVolt_V>"
  Bus Selector/4 -> essTsignalRange/2(signalValue)  "<essTemp_C>"
  " "/1 -> Bus Creator/2  "BMS_contactorsFailed_SigValid"
  Bus Selector/3 -> Sum/2  "<hvBusVolt_V>"
  Bus Creator/1 -> ESS_SigDiag/1  "ESS_SignalDiag"
  Sum/1 -> Abs/1
  Constant/1 -> essTsignalRange/1(clearFaults)
  Abs/1 -> " "/1
  essTsignalRange/1(essTempRange) -> essTsignalValidity_Check/1(In1), Bus Creator/5  "essTempRange[0_4]"
  essTsignalValidity_Check/1(Out1) -> Bus Creator/4  "BMS_essTemp_[degC]_SigValid"
  Bus Selector/5 -> essSOC_0_1Range/2(signalValue)  "<essSOC_0_1>"
  Constant1/1 -> essSOC_0_1Range/1(clearFaults)
  essSOCValidity_Check/1(Out1) -> Bus Creator/6  "BMS_essSOC_0_1_SigValid"
  Bus Selector/6 -> Interval Test/1  "<essCur_A>"
  Interval Test/1 -> Bus Creator/8  "essCur_A_SigValid"
  Bus Selector/7 -> Interval Test1/1  "<BMS_gdf>"
  Interval Test1/1 -> Bus Creator/9  "BMSgdf_0_1"
  essSOC_0_1Range/1(essSOCRange) -> Bus Creator/7, essSOCValidity_Check/1(In1)

== system P2_SIL_Model_Diag/Controller/HSC/Camaro Fault Detection/Signal Diagnostic/Engine Signal Diagnostic ==
  note: Engine_Temp:
      | Normal range: <100
      | above max:>120
      | Limited range: 100-120
  Sensors1 : Inport
  Bus Creator : BusCreator  Inputs=9
  Bus Selector : BusSelector  OutputSignals=ECM_Conv. ECMrollingAliveCnt [123],ECM_Conv. ECMTrqCmd_Nm,ECM_Conv.EngActStdyStTorq_Nm,ECM_Conv.EngineSpeed_rpm,ECM_Conv.Engine_Temp[DegC],ECM_Conv.EngRunAtv
  Constant1 : Constant
  EngTempValidity_Check : Subsystem  AncestorBlock=Diagnostic/Camaro Diagnostic/Signal Diagnostic/ESS Signal Diagnostic/essTsignalValidity_Check
  Engine_Temp[DegC] : Stateflow chart  TreatAsAtomicUnit=on
  Interval Test : simulink/Logic and Bit Operations/Interval Test  IntervalClosedRight=on  uplimit=233  IntervalClosedLeft=on  lowlimit=0  OutDataTypeStr=boolean
  Interval Test1 : simulink/Logic and Bit Operations/Interval Test  IntervalClosedRight=on  uplimit=6500  IntervalClosedLeft=on  lowlimit=0  OutDataTypeStr=boolean
  Interval Test2 : simulink/Logic and Bit Operations/Interval Test  IntervalClosedRight=on  uplimit=233  IntervalClosedLeft=on  lowlimit=0  OutDataTypeStr=boolean
  Interval Test3 : simulink/Logic and Bit Operations/Interval Test  IntervalClosedRight=on  uplimit=1  IntervalClosedLeft=on  lowlimit=0  OutDataTypeStr=boolean
  Rolling Alive Counter Detection1 : Subsystem  AncestorBlock=Diagnostic/Camaro Diagnostic/Signal Diagnostic/Motor Signal Diagnostic/Rolling Alive Counter Detection
  Engine_SigDiag : Outport
  wires:
  Sensors1/1 -> Bus Selector/1
  Bus Selector/1 -> Rolling Alive Counter Detection1/1(In1)  "< ECMrollingAliveCnt [123]>"
  Rolling Alive Counter Detection1/1(Out1) -> Bus Creator/1  "ECMRollingAliveActive"
  Bus Selector/2 -> Bus Creator/2, Interval Test/1  "< ECMTrqCmd_Nm>"
  Interval Test/1 -> Bus Creator/3  "engTrqCmdRecvd_SigValid"
  Bus Creator/1 -> Engine_SigDiag/1  "Engine_SignalDiag"
  Bus Selector/4 -> Interval Test1/1  "<EngineSpeed_rpm>"
  Interval Test1/1 -> Bus Creator/6  "Engine_Speed_rpm_SigValid"
  Bus Selector/3 -> Bus Creator/5, Interval Test2/1  "<EngActStdyStTorq_Nm>"
  Interval Test2/1 -> Bus Creator/4  "EngActStdyStTorq_SigValid"
  Bus Selector/5 -> Engine_Temp[DegC]/2(Engine_Temp_DegC)  "<Engine_Temp[DegC]>"
  Bus Selector/6 -> Interval Test3/1  "<EngRunAtv>"
  Interval Test3/1 -> Bus Creator/9  "EngRunAtValid"
  Constant1/1 -> Engine_Temp[DegC]/1(clearFaults)
  Engine_Temp[DegC]/1(EngTempRange) -> EngTempValidity_Check/1(In1), Bus Creator/8  "Eng_TempRange[123]"
  EngTempValidity_Check/1(Out1) -> Bus Creator/7  "Eng_TempValid"

== system P2_SIL_Model_Diag/Controller/HSC/Camaro Fault Detection/Signal Diagnostic/Motor Signal Diagnostic ==
  note: 1 = Forward
      | 0 = 'Reverse' if inverter enabled  & 'Stopped' if inverter is disabled
  note: MCU : Signal Diagnostic
  note: Temperature Range check :
      | 0 = below normal operation (<-40)
      | 1 = low range (<0 - >-30)
      | 2 = normal range (-31 -80 C)
      | 3= high range (>80)
      | 4= above max value allowed (>100)
  Sensors1 : Inport
  Bus Creator : BusCreator  Inputs=18
  Bus Selector : BusSelector  OutputSignals=MCU_Conv. MCUrollingAliveCnt [123],MCU_Conv. MCUTemp_C,MCU_Conv.Motor_Temp_C,MCU_Conv.MCUTrqCmd_Nm,MCU_Conv.Torq_Feedback_Nm,MCU_Conv.MotorSpeed_rpm,MCU_Conv.Direction_Command_0_1,MCU_Conv.Direction_feedback_0_1,MCU_Conv.Inverter_enable_state_0_1,MCU_Conv.DC_Bus_Voltage_V
  Constant : Constant
  Constant1 : Constant
  Constant2 : Constant  Value=50
  Interval Test : simulink/Logic and Bit Operations/Interval Test  IntervalClosedRight=on  uplimit=350  IntervalClosedLeft=on  lowlimit=-350  OutDataTypeStr=boolean
  Interval Test1 : simulink/Logic and Bit Operations/Interval Test  IntervalClosedRight=on  uplimit=8000  IntervalClosedLeft=on  lowlimit=0  OutDataTypeStr=boolean
  Interval Test2 : simulink/Logic and Bit Operations/Interval Test  IntervalClosedRight=on  uplimit=350  IntervalClosedLeft=on  lowlimit=-350  OutDataTypeStr=boolean
  Interval Test3 : simulink/Logic and Bit Operations/Interval Test  IntervalClosedRight=on  uplimit=1  IntervalClosedLeft=on  lowlimit=0  OutDataTypeStr=boolean
  Interval Test4 : simulink/Logic and Bit Operations/Interval Test  IntervalClosedRight=on  uplimit=1  IntervalClosedLeft=on  lowlimit=0  OutDataTypeStr=boolean
  Interval Test5 : simulink/Logic and Bit Operations/Interval Test  IntervalClosedRight=on  uplimit=1  IntervalClosedLeft=on  lowlimit=0  OutDataTypeStr=boolean
  Interval Test6 : simulink/Logic and Bit Operations/Interval Test  IntervalClosedRight=on  uplimit=390  IntervalClosedLeft=on  lowlimit=-390  OutDataTypeStr=boolean
  Rolling Alive Counter Detection : Subsystem
  Subsystem : Subsystem
  Subsystem1 : Subsystem
  Terminator : Terminator
  Motor_SigDiag : Outport
  wires:
  Sensors1/1 -> Bus Selector/1
  Bus Selector/1 -> Rolling Alive Counter Detection/1(In1)  "< MCUrollingAliveCnt [123]>"
  Rolling Alive Counter Detection/1(Out1) -> Bus Creator/1  "MCURollingAliveActive"
  Bus Creator/1 -> Motor_SigDiag/1  "Motor_SignalDiag"
  Bus Selector/6 -> Interval Test1/1  "<MotorSpeed_rpm>"
  Interval Test1/1 -> Bus Creator/10  "Motor_Speed_rpm_SigValid"
  Interval Test/1 -> Bus Creator/6  "Motor_TrqCmd_Nm_SigValid"
  Bus Selector/4 -> Interval Test/1, Bus Creator/7  "<MCUTrqCmd_Nm>"
  Bus Selector/5 -> Interval Test2/1, Bus Creator/9  "<Torq_Feedback_Nm>"
  Interval Test2/1 -> Bus Creator/8  "Torq_Feedback_Nm_SigValid"
  Bus Selector/7 -> Interval Test3/1, Bus Creator/12  "<Direction_Command_0_1>"
  Interval Test3/1 -> Bus Creator/11  "Direction_Command_SigValid"
  Bus Selector/8 -> Interval Test4/1, Bus Creator/14  "<Direction_feedback_0_1>"
  Bus Selector/9 -> Bus Creator/16, Interval Test5/1  "<Inverter_enable_state_0_1>"
  Interval Test4/1 -> Bus Creator/13  "Direction_feedback_SigValid"
  Interval Test5/1 -> Bus Creator/15  "Inverter_enable_state_SigValid"
  Constant/1 -> Subsystem/1(ClearFault)
  Subsystem/1(MCUTemp_degC_SigValid) -> Bus Creator/2
  Constant1/1 -> Subsystem1/1(ClearFault)
  Bus Selector/3 -> Subsystem1/2(In2)  "<Motor_Temp_C>"
  Subsystem1/1(MotorTemp_degC_SigValid) -> Bus Creator/4
  Subsystem1/2(MotorTempRange) -> Bus Creator/5
  Bus Selector/10 -> Bus Creator/18, Interval Test6/1  "<DC_Bus_Voltage_V>"
  Interval Test6/1 -> Bus Creator/17  "DC_Bus_Voltage_SigValid"
  Subsystem/2(MCUTempRange) -> Bus Creator/3
  Bus Selector/2 -> Terminator/1  "< MCUTemp_C>"
  Constant2/1 -> Subsystem/2(In2)

== system P2_SIL_Model_Diag/Controller/HSC/Camaro Fault Detection/Signal Diagnostic/Transmission Signal Diagnostic ==
  note: TransEstGear
      | 0 : Not Supported
      | 1 : First Gear
      | 2 : Second Gear
      | 3 : Third Gear
      | 4 : Fourth Gear
      | 5 : Fifth Gear
      | 6 : Sixth Gear
      | 7 : Seventh Gear
      | 8 : Eight Gear
      | 10: EVT Mode 1
      | 11: EVT Mode 2
      | 12: CVT Forward Gear
      | 13: Neutral Gear
      | 14: Reverse Gear
      | 15: Park Gear
  note: Lever Position:
      | 1 P
      | 2 R
      | 3 N
      | 4 D
      | 0: L
  Sensors1 : Inport
  Bus Creator : BusCreator  Inputs=4
  Bus Selector : BusSelector  OutputSignals=TCM_Conv.TCMrollingAliveCnt [123],TCM_Conv. LvrPosTrnsShft,TCM_Conv.TransEstGear,TCM_Conv.LockupCmd_0_1
  Interval Test : simulink/Logic and Bit Operations/Interval Test  IntervalClosedRight=on  uplimit=4  IntervalClosedLeft=on  lowlimit=1  OutDataTypeStr=boolean
  Interval Test1 : simulink/Logic and Bit Operations/Interval Test  IntervalClosedRight=on  uplimit=15  IntervalClosedLeft=on  lowlimit=0  OutDataTypeStr=boolean
  Interval Test2 : simulink/Logic and Bit Operations/Interval Test  IntervalClosedRight=on  uplimit=1  IntervalClosedLeft=on  lowlimit=0  OutDataTypeStr=boolean
  Rolling Alive Counter Detection : Subsystem  AncestorBlock=Diagnostic/Camaro Diagnostic/Signal Diagnostic/Motor Signal Diagnostic/Rolling Alive Counter Detection
  Out2 : Outport
  wires:
  Sensors1/1 -> Bus Selector/1
  Bus Selector/1 -> Rolling Alive Counter Detection/1(In1)  "<TCMrollingAliveCnt [123]>"
  Rolling Alive Counter Detection/1(Out1) -> Bus Creator/1  "TCMRollingAliveActive_SigValid"
  Bus Creator/1 -> Out2/1
  Bus Selector/2 -> Interval Test/1  "< LvrPosTrnsShft>"
  Bus Selector/3 -> Interval Test1/1  "<TransEstGear>"
  Bus Selector/4 -> Interval Test2/1  "<LockupCmd_0_1>"
  Interval Test/1 -> Bus Creator/2  "LvrPosTrnsShft_SigValid"
  Interval Test1/1 -> Bus Creator/3  "TransEstGear_SigValid"
  Interval Test2/1 -> Bus Creator/4  "LockupCmd_SigValid"
